simulink model "Bands1"  (R2018a)
settings: Solver=VariableStepAuto  StartTime=0.0  StopTime=0.001  RelTol=1e-3
undefined symbols (not defined in the file): fdesignblkfcn, G1, gcbh, get, T
libraries: dspsrcs4 x1, dspxfrm3 x1, dspobslib x1
settings Model: Creator=Daniel  LastModifiedBy=Daniel

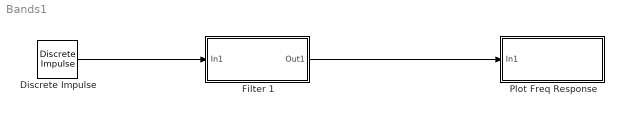
== system Bands1 ==
  Discrete Impulse : dspsrcs4/Discrete  Impulse  Delay=0  SampleTime=T  FrameSample=128  OutputFrames=off  dataType=double  isSigned=on  wordLen=16  udDataType=sfix(16)  fracBitsMode=Best precision  numFracBits=15  OutDataTypeStr=double  LastOutDataTypeStr=double
  Filter 1 : Subsystem
  Plot Freq Response : Subsystem
  wires:
  Discrete Impulse/1 -> Filter 1/1(In1)
  Filter 1/1(Out1) -> Plot Freq Response/1(In1)

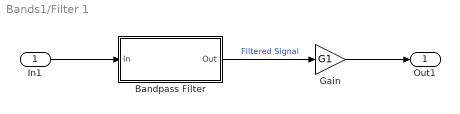
== system Bands1/Filter 1 ==
  In1 : Inport
  Bandpass Filter : Subsystem  DialogController=fdesignblkfcn  InitFcn=fdesignblkfcn(gcbh, {'InitFcn'});  mask(Bandpass Filter){}
      mask help: Design a bandpass filter
      settings: CopyFcn=fdesignblkfcn(gcbh, {'CopyFcn'});
      mask Help: helpview(mapfilelocation('dsp'), 'dspbandpassfilter');
      mask Display: disp('Bandpass');
  Gain : Gain  Gain=G1
  Out1 : Outport
  wires:
  Bandpass Filter/1(Out) -> Gain/1  "Filtered Signal"
  In1/1 -> Bandpass Filter/1(In)
  Gain/1 -> Out1/1

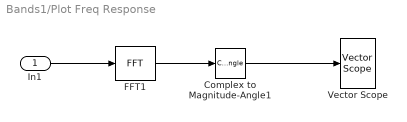
== system Bands1/Plot Freq Response ==
  In1 : Inport
  Complex to Magnitude-Angle1 : ComplexToMagnitudeAngle  Output=Magnitude
  FFT1 : dspxfrm3/FFT  FFTImplementation=Auto  CompMethod=Table lookup  TableOpt=NEW  TableOptActive=Speed  BitRevOrder=off  Normalize=off  InheritFFTLength=on  FFTLength=64  WrapInput=on  roundingMode=Floor  overflowMode=off  firstCoeffDataTypeStr=Inherit: Same word length as input  firstCoeffLastDataTypeStr=Inherit: Same word length as input  outputMin=[]  outputMax=[]
  Vector Scope : dspobslib/Vector Scope  ScopeProperties=off  Domain=Frequency  HorizSpan=1  DisplayProperties=off  AxisGrid=on  Memory=off  FrameNumber=off  AxisLegend=off  AxisZoom=off  OpenScopeAtSimStart=on  OpenScopeImmediately=off  FigPos=get(0,'defaultfigureposition')  AxisProperties=on  XUnits=Hertz  XRange=[0...Fs/2]  InheritXIncr=on  XIncr=1  XLabel=Samples  XLimit=Auto  XMin=0  XMax=1  XStart=0  YUnits=dB  YLabel=|Magnitude (dB)|  LineProperties=off  XAxisParamsVer=6.9
      settings: SourceProductName=DSP System Toolbox  SourceProductBaseCode=DS  YMin=0.0723692553519949  YMax=69.3188381671759
  wires:
  In1/1 -> FFT1/1
  FFT1/1 -> Complex to Magnitude-Angle1/1
  Complex to Magnitude-Angle1/1 -> Vector Scope/1

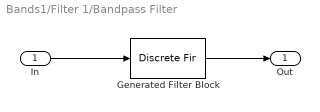
== system Bands1/Filter 1/Bandpass Filter ==
  In : Inport
  Generated Filter Block : DiscreteFir  Tag=BlockMethodSubSystem  Coefficients=[0.0178974290421398917 -0.0154023645825985753 -0.0135117522966385264 -0.00346743039279297921 -0.0140131602279785251 0.00254852418665821485 -0.0134572168089668997 0.000324499679083851934 -0.00772012234546977719 -0.00673636483835179847 -0.00218012238033685364 -0.0100772161008637687 -0.00397604673120863835 -0.00552052308204037997 -0.0119023843401352119 0.000782658282824639779 -0.0164372958684521168 -0.000734221542822768251 -0.0112348596615164213 -0.0105890209397578126 -0.00225628929859128134 -0.0178838277331088286 -0.0017893174684224689 -0.0131765299729471094 -0.0127928324303829399 -0.00165420402169025099 -0.0230245384226856961 0.00108076329694036942 -0.0187503825846339171 -0.0117064182520684561 -0.00331937020703018367 -0.0266367204167449849 0.0035906574400060569 -0.0240197267630196561 -0.0107436679241715901 -0.00343180388140861166 -0.0327586317402937324 0.0104438559305362211 -0.0336868658531658607 -0.00580354191623811549 -0.00431216319204353639 -0.0415814804909801425 0.024947805529904131 -0.0529645754809640879 0.00780432330552301677 -0.00440426053693279348 -0.0691021439889363542 0.0888921836054180764 -0.16261022991752605 0.164196114634056645 0.795274140970088306 0.164196114634056645 -0.16261022991752605 0.0888921836054180764 -0.0691021439889363542 -0.00440426053693279348 0.00780432330552301677 -0.0529645754809640879 0.024947805529904131 -0.0415814804909801425 -0.00431216319204353639 -0.00580354191623811549 -0.0336868658531658607 0.0104438559305362211 -0.0327586317402937324 -0.00343180388140861166 -0.0107436679241715901 -0.0240197267630196561 0.0035906574400060569 -0.0266367204167449849 -0.00331937020703018367 -0.0117064182520684561 -0.0187503825846339171 0.00108076329694036942 -0.0230245384226856961 -0.00165420402169025099 -0.0127928324303829399 -0.0131765299729471094 -0.0017893174684224689 -0.0178838277331088286 -0.00225628929859128134 -0.0105890209397578126 -0.0112348596615164213 -0.000734221542822768251 -0.0164372958684521168 0.000782658282824639779 -0.0119023843401352119 -0.00552052308204037997 -0.00397604673120863835 -0.0100772161008637687 -0.00218012238033685364 -0.00673636483835179847 -0.00772012234546977719 0.000324499679083851934 -0.0134572168089668997 0.00254852418665821485 -0.0140131602279785251 -0.00346743039279297921 -0.0135117522966385264 -0.0154023645825985753 0.0178974290421398917]  InputProcessing=Columns as channels (frame based)
  Out : Outport
  wires:
  In/1 -> Generated Filter Block/1
  Generated Filter Block/1 -> Out/1
